simulink model "torqueRequest_plausibility"  (R2024b)
settings: Solver=FixedStepAuto  StartTime=0.0  StopTime=20  RelTol=1e-3
settings Model: Creator=aayan  LastModifiedBy=aayan
settings ConfigComp: CovEnable=on  RecordCoverage=on  CovMetricSettings=dcmwe  CovModelRefEnable=on

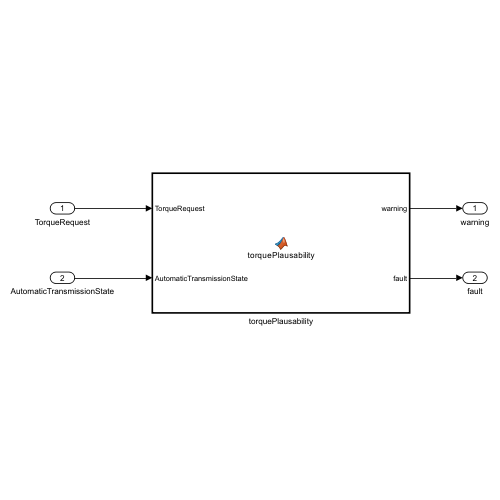
[thumbnail: Simulink's stored preview of the top-level diagram]
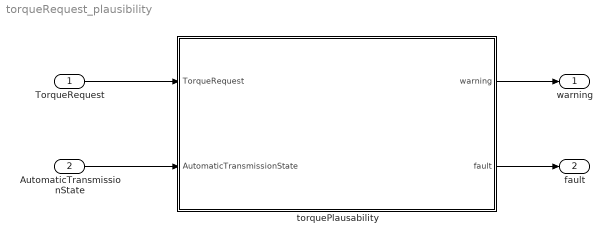
== system torqueRequest_plausibility ==
  TorqueRequest : Inport  OutDataTypeStr=single
  AutomaticTransmissionState : Inport  Port=2  OutDataTypeStr=Enum: TransmissionState
  torquePlausability : MATLAB Function  TreatAsAtomicUnit=on
  warning : Outport  OutDataTypeStr=boolean
  fault : Outport  Port=2  OutDataTypeStr=boolean
  wires:
  torquePlausability/1(warning) -> warning/1
  torquePlausability/2(fault) -> fault/1
  TorqueRequest/1 -> torquePlausability/1(TorqueRequest)
  AutomaticTransmissionState/1 -> torquePlausability/2(AutomaticTransmissionState)

== matlab function torqueRequest_plausibility/torquePlausability ==
  data: TorqueRequest input; warning output; fault output; AutomaticTransmissionState input
function [warning, fault] = torquePlausability(TorqueRequest,AutomaticTransmissionState)
% initialization
warning = boolean(0);
fault = boolean(0);

if (TorqueRequest > 80 || TorqueRequest < -80 )
    warning = boolean(1);
    fault = boolean(1);
elseif((AutomaticTransmissionState ~= TransmissionState.Reverse && AutomaticTransmissionState ~= TransmissionState.Brake ) && TorqueRequest < 0 )
    warning = boolean(1);
    fault = boolean(1); 
elseif ((AutomaticTransmissionState ~= TransmissionState.Drive && AutomaticTransmissionState ~= TransmissionState.Brake) && TorqueRequest> 0)
    warning = boolean(1);
    fault = boolean(1);
end
